simulink model "EarlyReturn6_2018a"  (R2018a)
settings: Solver=VariableStepAuto  StartTime=0.0  StopTime=0.1  RelTol=1e-3
settings Model: Creator=BEAR  LastModifiedBy=apple

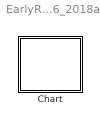
== system EarlyReturn6_2018a ==
  Chart : Stateflow chart  TreatAsAtomicUnit=on

== stateflow chart EarlyReturn6_2018a/Chart ==
  settings: updateMethod=DISCRETE  sampleTime=0.1
  state A
    en: fprintf("en_A")
    ex: fprintf("ex_A")
    state A1
      en: fprintf("en_A1")
      ex: fprintf("ex_A1")
    state A2
      en: fprintf("en_A2")
      ex: fprintf("ex_A2")
    (default) -> A1
    A1 -> A2 : /{E;fprintf("ta")}
  (default) -> A
  A -> A : E{fprintf("loop")}
  events: E local FUNCTION_CALL_EVENT
